simulink model "backstepping_and_CT"  (R2020b)
settings: Solver=ode23t  StartTime=0.0  StopTime=30  RelTol=1e-3
InitFcn:
  | parametersUR5_BACKSTEPPING
StopFcn:
  | show_results
values from neighbouring files (symbols this model uses):
  init_config = [0,-55.5,-131,-2.5,20,105]'*pi/180    [UR5_LI_SLOTINE.m]    (also in parametersUR5_ADAPTIVE_BACKSTEPPING.m = [0,-37,-110,-2.5,-1,55]'*pi/180; parametersUR5_BACKSTEPPING.m = [0,-37,-110,-2.5,-1,55]'*pi/180)
  m1 = ur5.links(1,1).m    [UR5_LI_SLOTINE.m]    (also in parametersUR5_ADAPTIVE_BACKSTEPPING.m; parametersUR5_BACKSTEPPING.m)
  m2 = ur5.links(1,2).m    [UR5_LI_SLOTINE.m]    (also in parametersUR5_ADAPTIVE_BACKSTEPPING.m; parametersUR5_BACKSTEPPING.m)
  m3 = ur5.links(1,3).m    [UR5_LI_SLOTINE.m]    (also in parametersUR5_ADAPTIVE_BACKSTEPPING.m; parametersUR5_BACKSTEPPING.m)
  m4 = ur5.links(1,4).m    [UR5_LI_SLOTINE.m]    (also in parametersUR5_ADAPTIVE_BACKSTEPPING.m; parametersUR5_BACKSTEPPING.m)
  m5 = ur5.links(1,5).m    [UR5_LI_SLOTINE.m]    (also in parametersUR5_ADAPTIVE_BACKSTEPPING.m; parametersUR5_BACKSTEPPING.m)
  m6 = ur5.links(1,6).m    [UR5_LI_SLOTINE.m]    (also in parametersUR5_ADAPTIVE_BACKSTEPPING.m; parametersUR5_BACKSTEPPING.m)
  Ts = 1/100    (= 0.01)    [UR5_LI_SLOTINE.m]    (also in parametersUR5_ADAPTIVE_BACKSTEPPING.m; parametersUR5_BACKSTEPPING.m)
libraries: simulink x2
settings Model: Creator=marym  LastModifiedBy=stefa
settings DebuggingCC: SFMachineParentedDataDiag=error

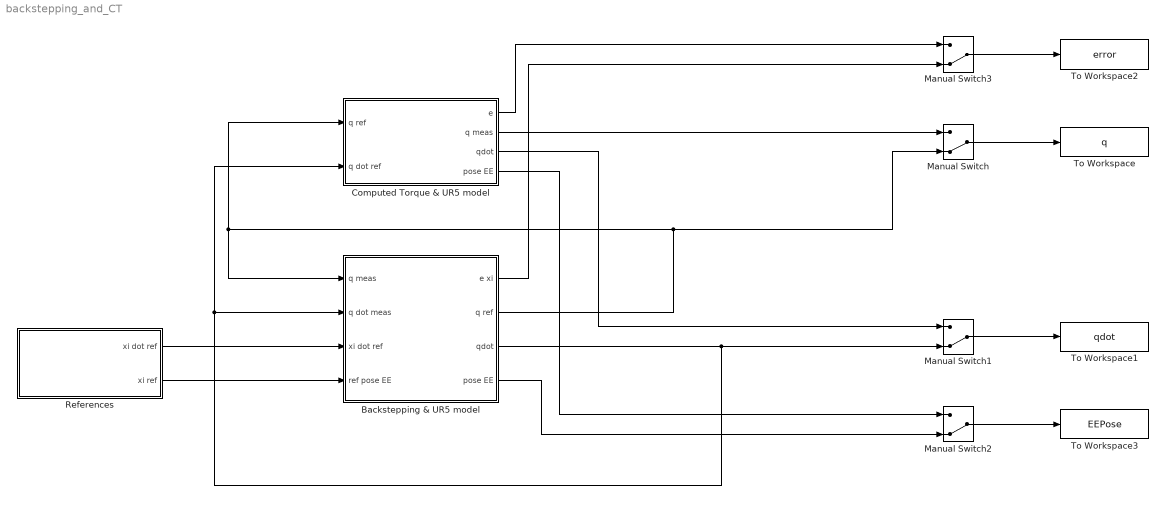
== system backstepping_and_CT ==
  Backstepping & UR5 model : Subsystem
  Computed Torque & UR5 model : Subsystem
  Manual Switch{,1..3} (4 alike) : ManualSwitch  CurrentSetting=0
  References : Subsystem
  To Workspace : ToWorkspace  VariableName=q  SaveFormat=Timeseries  SampleTime=Ts
  To Workspace1 : ToWorkspace  VariableName=qdot  SaveFormat=Timeseries  SampleTime=Ts
  To Workspace2 : ToWorkspace  VariableName=error  SaveFormat=Timeseries  SampleTime=Ts
  To Workspace3 : ToWorkspace  VariableName=EEPose  SaveFormat=Timeseries  SampleTime=Ts
  wires:
  Manual Switch/1 -> To Workspace/1
  Manual Switch1/1 -> To Workspace1/1
  Manual Switch2/1 -> To Workspace3/1
  Manual Switch3/1 -> To Workspace2/1
  Backstepping & UR5 model/3(qdot) -> Computed Torque & UR5 model/2(q dot ref), Backstepping & UR5 model/2(q dot meas), Manual Switch1/2
  Backstepping & UR5 model/2(q ref) -> Manual Switch/2, Computed Torque & UR5 model/1(q ref), Backstepping & UR5 model/1(q meas)
  References/1(xi dot ref) -> Backstepping & UR5 model/3(xi dot ref)
  References/2(xi ref) -> Backstepping & UR5 model/4(ref pose EE)
  Backstepping & UR5 model/1(e xi) -> Manual Switch3/2
  Backstepping & UR5 model/4(pose EE) -> Manual Switch2/2
  Computed Torque & UR5 model/1(e) -> Manual Switch3/1
  Computed Torque & UR5 model/2(q meas) -> Manual Switch/1
  Computed Torque & UR5 model/3(qdot) -> Manual Switch1/1
  Computed Torque & UR5 model/4(pose EE) -> Manual Switch2/1

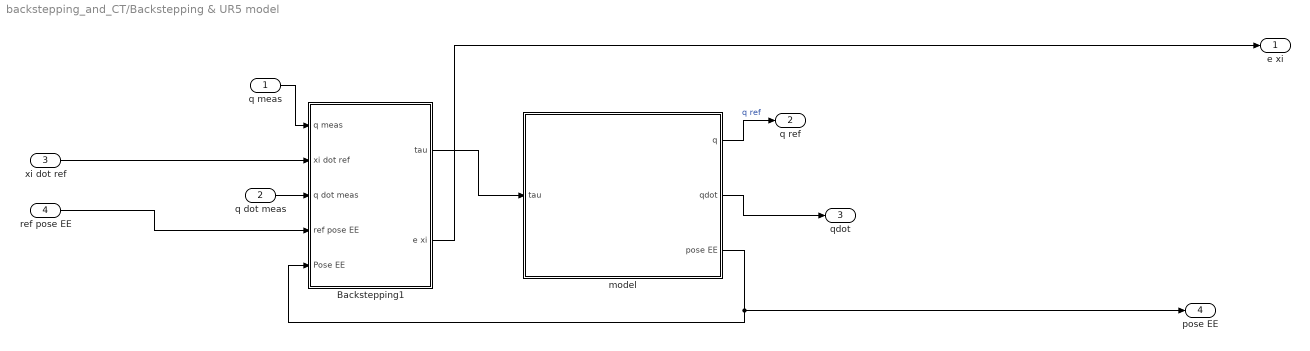
== system backstepping_and_CT/Backstepping & UR5 model ==
  q meas : Inport
  q dot meas : Inport  Port=2
  xi dot ref : Inport  Port=3
  ref pose EE : Inport  Port=4
  Backstepping1 : Subsystem
  model : Subsystem
  e xi : Outport
  q ref : Outport  Port=2
  qdot : Outport  Port=3
  pose EE : Outport  Port=4
  wires:
  model/1(q) -> q ref/1  "q ref"
  Backstepping1/2(e xi) -> e xi/1
  ref pose EE/1 -> Backstepping1/4(ref pose EE)
  Backstepping1/1(tau) -> model/1(tau)
  model/3(pose EE) -> pose EE/1, Backstepping1/5(Pose EE)
  model/2(qdot) -> qdot/1
  q meas/1 -> Backstepping1/1(q meas)
  q dot meas/1 -> Backstepping1/3(q dot meas)
  xi dot ref/1 -> Backstepping1/2(xi dot ref)

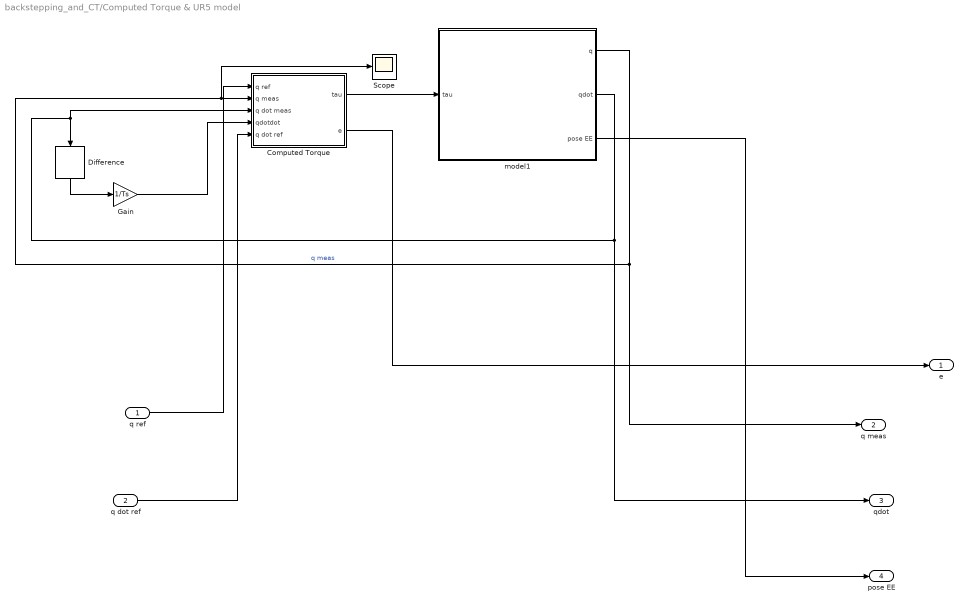
== system backstepping_and_CT/Computed Torque & UR5 model ==
  q ref : Inport
  q dot ref : Inport  Port=2
  Computed Torque : Subsystem
  Difference : simulink/Discrete/Difference  ICPrevInput=0.0  OutMin=[]  OutMax=[]  OutDataType=fixdt(1, 16)  OutScaling=2^-10  DoSatur=off
  Gain : Gain  Gain=1/Ts
  Scope : Scope
  model1 : Subsystem
  e : Outport
  q meas : Outport  Port=2
  qdot : Outport  Port=3
  pose EE : Outport  Port=4
  wires:
  model1/3(pose EE) -> pose EE/1
  model1/1(q) -> q meas/1, Scope/1, Computed Torque/2(q meas)  "q meas"
  Computed Torque/1(tau) -> model1/1(tau)
  model1/2(qdot) -> qdot/1, Computed Torque/3(q dot meas), Difference/1
  q ref/1 -> Computed Torque/1(q ref)
  Difference/1 -> Gain/1
  Gain/1 -> Computed Torque/4(qdotdot)
  q dot ref/1 -> Computed Torque/5(q dot ref)
  Computed Torque/2(e) -> e/1

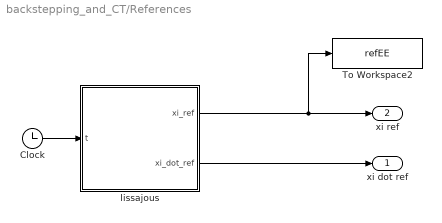
== system backstepping_and_CT/References ==
  Clock : Clock
  To Workspace2 : ToWorkspace  VariableName=refEE  SaveFormat=Timeseries  SampleTime=Ts
  lissajous : MATLAB Function  TreatAsAtomicUnit=on
  xi dot ref : Outport
  xi ref : Outport  Port=2
  wires:
  Clock/1 -> lissajous/1(t)
  lissajous/1(xi_ref) -> To Workspace2/1, xi ref/1
  lissajous/2(xi_dot_ref) -> xi dot ref/1

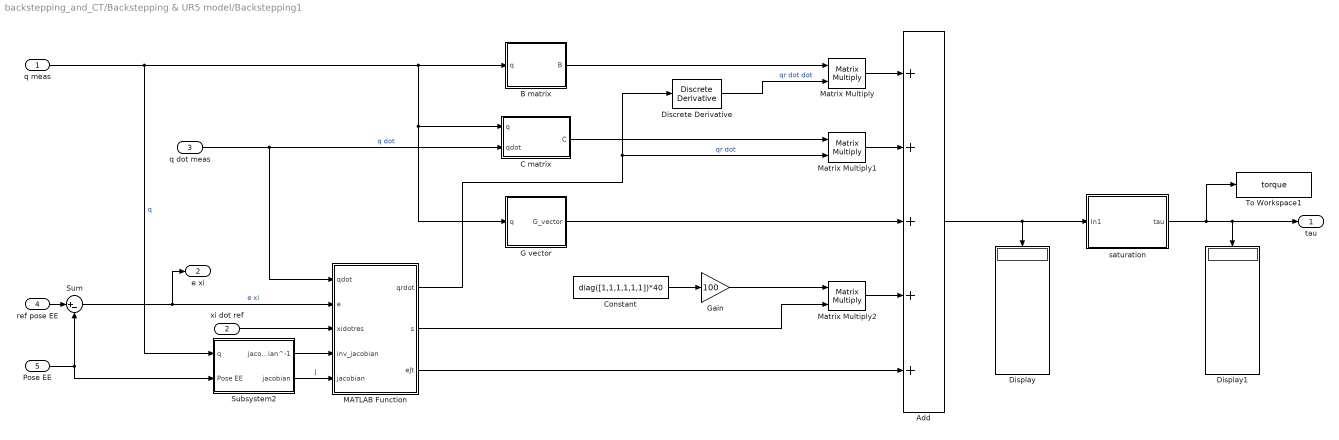
== system backstepping_and_CT/Backstepping & UR5 model/Backstepping1 ==
  q meas : Inport
  xi dot ref : Inport  Port=2
  q dot meas : Inport  Port=3
  ref pose EE : Inport  Port=4
  Pose EE : Inport  Port=5
  Add : Sum  Inputs=+++++
  B matrix : MATLAB Function  TreatAsAtomicUnit=on
  C matrix : MATLAB Function  TreatAsAtomicUnit=on
  Constant : Constant  Value=diag([1,1,1,1,1,1])*40
  Discrete Derivative : simulink/Discrete/Discrete Derivative  gainval=1.0  ICPrevScaledInput=0.0  OutMin=[]  OutMax=[]  OutDataType=fixdt(1, 16)  OutScaling=2^-10  DoSatur=off
  Display : Display
  Display1 : Display
  G vector : MATLAB Function  TreatAsAtomicUnit=on
  Gain : Gain  Gain=100
  MATLAB Function : MATLAB Function  TreatAsAtomicUnit=on
  Matrix Multiply : Product  Multiplication=Matrix(*)
  Matrix Multiply1 : Product  Multiplication=Matrix(*)
  Matrix Multiply2 : Product  Multiplication=Matrix(*)
  Subsystem2 : Subsystem
  Sum : Sum  Inputs=|+-
  To Workspace1 : ToWorkspace  VariableName=torque  SaveFormat=Timeseries  SampleTime=Ts
  saturation : Subsystem
  tau : Outport
  e xi : Outport  Port=2
  wires:
  Add/1 -> Display/1, saturation/1(In1)
  Matrix Multiply/1 -> Add/1
  Matrix Multiply1/1 -> Add/2
  B matrix/1(B) -> Matrix Multiply/1
  C matrix/1(C) -> Matrix Multiply1/1
  q meas/1 -> G vector/1(q), C matrix/1(q), B matrix/1(q), Subsystem2/1(q)  "q"
  G vector/1(G_vector) -> Add/3
  Discrete Derivative/1 -> Matrix Multiply/2  "qr dot dot"
  MATLAB Function/1(qrdot) -> Matrix Multiply1/2, Discrete Derivative/1  "qr dot"
  q dot meas/1 -> MATLAB Function/1(qdot), C matrix/2(qdot)  "q dot"
  ref pose EE/1 -> Sum/1
  Pose EE/1 -> Sum/2, Subsystem2/2(Pose EE)
  Sum/1 -> e xi/1, MATLAB Function/2(e)  "e xi"
  Subsystem2/1(jacobian^-1) -> MATLAB Function/4(inv_jacobian)
  MATLAB Function/3(eJt) -> Add/5
  Subsystem2/2(jacobian) -> MATLAB Function/5(jacobian)  "J"
  MATLAB Function/2(s) -> Matrix Multiply2/2
  Matrix Multiply2/1 -> Add/4
  Constant/1 -> Gain/1
  xi dot ref/1 -> MATLAB Function/3(xidotres)
  Gain/1 -> Matrix Multiply2/1
  saturation/1(tau) -> tau/1, Display1/1, To Workspace1/1

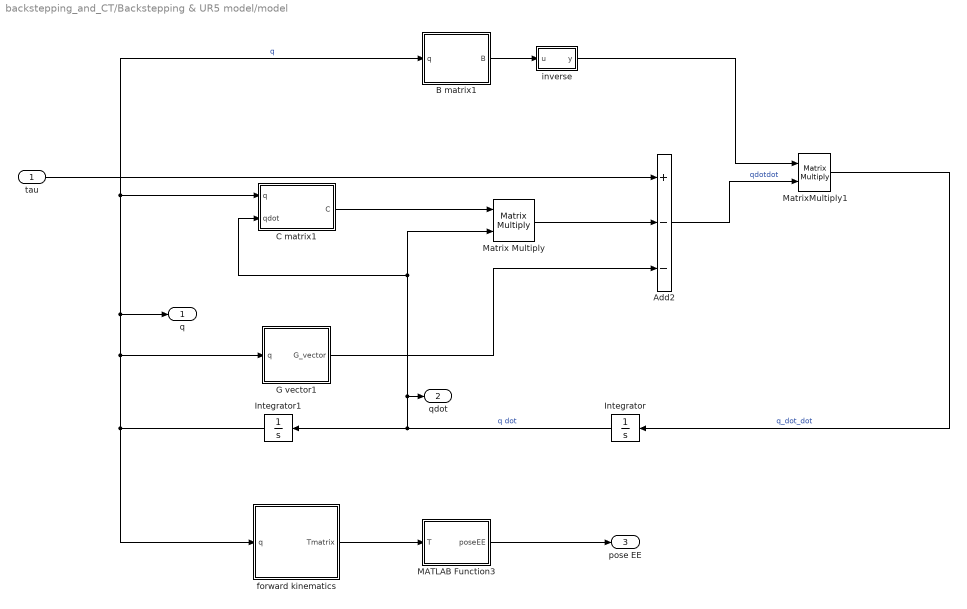
== system backstepping_and_CT/Backstepping & UR5 model/model ==
  tau : Inport
  Add2 : Sum  Inputs=+--
  B matrix1 : MATLAB Function  TreatAsAtomicUnit=on
  C matrix1 : MATLAB Function  TreatAsAtomicUnit=on
  G vector1 : MATLAB Function  TreatAsAtomicUnit=on
  Integrator : Integrator  InitialCondition=[0,0,0,0,0,0]'
  Integrator1 : Integrator  InitialCondition=init_config
  MATLAB Function3 : MATLAB Function  TreatAsAtomicUnit=on
  Matrix Multiply : Product  Multiplication=Matrix(*)
  MatrixMultiply1 : Product  Multiplication=Matrix(*)
  forward kinematics : MATLAB Function  TreatAsAtomicUnit=on
  inverse : MATLAB Function  TreatAsAtomicUnit=on
  q : Outport
  qdot : Outport  Port=2
  pose EE : Outport  Port=3
  wires:
  MatrixMultiply1/1 -> Integrator/1  "q_dot_dot"
  B matrix1/1(B) -> inverse/1(u)
  inverse/1(y) -> MatrixMultiply1/1
  tau/1 -> Add2/1
  Matrix Multiply/1 -> Add2/2
  C matrix1/1(C) -> Matrix Multiply/1
  Integrator/1 -> C matrix1/2(qdot), Matrix Multiply/2, qdot/1, Integrator1/1  "q dot"
  Integrator1/1 -> forward kinematics/1(q), G vector1/1(q), q/1, B matrix1/1(q), C matrix1/1(q)  "q"
  G vector1/1(G_vector) -> Add2/3
  Add2/1 -> MatrixMultiply1/2  "qdotdot"
  forward kinematics/1(Tmatrix) -> MATLAB Function3/1(T)
  MATLAB Function3/1(poseEE) -> pose EE/1

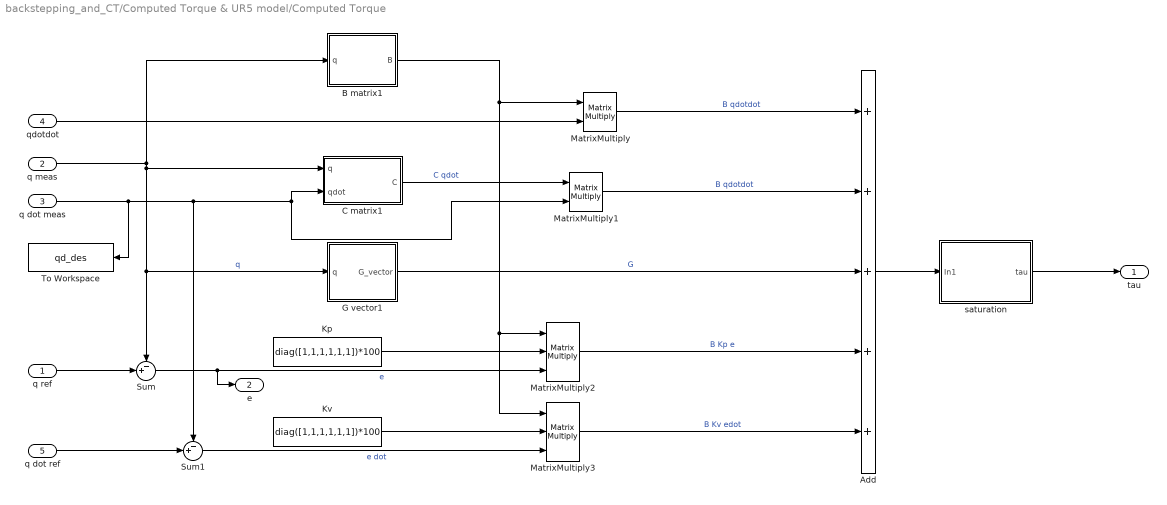
== system backstepping_and_CT/Computed Torque & UR5 model/Computed Torque ==
  q ref : Inport
  q meas : Inport  Port=2
  q dot meas : Inport  Port=3
  qdotdot : Inport  Port=4
  q dot ref : Inport  Port=5
  Add : Sum  Inputs=+++++
  B matrix1 : MATLAB Function  TreatAsAtomicUnit=on
  C matrix1 : MATLAB Function  TreatAsAtomicUnit=on
  G vector1 : MATLAB Function  TreatAsAtomicUnit=on
  Kp : Constant  Value=diag([1,1,1,1,1,1])*100
  Kv : Constant  Value=diag([1,1,1,1,1,1])*100
  MatrixMultiply : Product  Multiplication=Matrix(*)
  MatrixMultiply1 : Product  Multiplication=Matrix(*)
  MatrixMultiply2 : Product  Inputs=3  Multiplication=Matrix(*)
  MatrixMultiply3 : Product  Inputs=3  Multiplication=Matrix(*)
  Sum : Sum  Inputs=-+|
  Sum1 : Sum  Inputs=-+|
  To Workspace : ToWorkspace  VariableName=qd_des  SaveFormat=Timeseries  SampleTime=-1
  saturation : Subsystem
  tau : Outport
  e : Outport  Port=2
  wires:
  q meas/1 -> C matrix1/1(q), G vector1/1(q), Sum/1, B matrix1/1(q)  "q"
  MatrixMultiply/1 -> Add/1  "B qdotdot"
  B matrix1/1(B) -> MatrixMultiply3/1, MatrixMultiply2/1, MatrixMultiply/1
  q dot meas/1 -> To Workspace/1, Sum1/1, C matrix1/2(qdot), MatrixMultiply1/2
  C matrix1/1(C) -> MatrixMultiply1/1  "C qdot"
  G vector1/1(G_vector) -> Add/3  "G"
  q ref/1 -> Sum/2
  Sum/1 -> e/1, MatrixMultiply2/3  "e"
  MatrixMultiply2/1 -> Add/4  "B Kp e"
  q dot ref/1 -> Sum1/2
  Sum1/1 -> MatrixMultiply3/3  "e dot"
  MatrixMultiply3/1 -> Add/5  "B Kv edot"
  Kp/1 -> MatrixMultiply2/2
  Kv/1 -> MatrixMultiply3/2
  qdotdot/1 -> MatrixMultiply/2
  MatrixMultiply1/1 -> Add/2  "B qdotdot"
  Add/1 -> saturation/1(In1)
  saturation/1(tau) -> tau/1

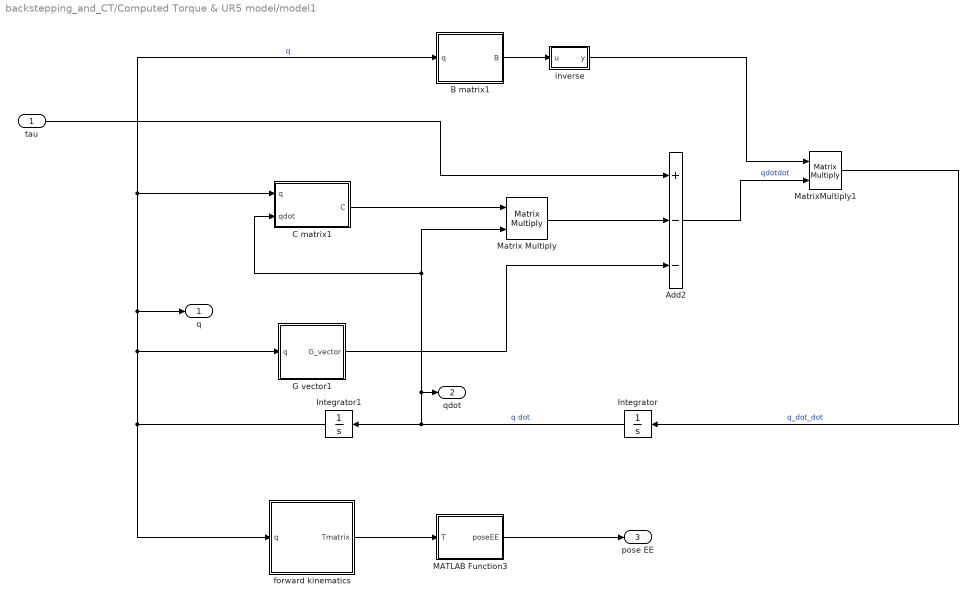
== system backstepping_and_CT/Computed Torque & UR5 model/model1 ==
  tau : Inport
  Add2 : Sum  Inputs=+--
  B matrix1 : MATLAB Function  TreatAsAtomicUnit=on
  C matrix1 : MATLAB Function  TreatAsAtomicUnit=on
  G vector1 : MATLAB Function  TreatAsAtomicUnit=on
  Integrator : Integrator  InitialCondition=[0,0,0,0,0,0]'
  Integrator1 : Integrator  InitialCondition=init_config
  MATLAB Function3 : MATLAB Function  TreatAsAtomicUnit=on
  Matrix Multiply : Product  Multiplication=Matrix(*)
  MatrixMultiply1 : Product  Multiplication=Matrix(*)
  forward kinematics : MATLAB Function  TreatAsAtomicUnit=on
  inverse : MATLAB Function  TreatAsAtomicUnit=on
  q : Outport
  qdot : Outport  Port=2
  pose EE : Outport  Port=3
  wires:
  MatrixMultiply1/1 -> Integrator/1  "q_dot_dot"
  B matrix1/1(B) -> inverse/1(u)
  inverse/1(y) -> MatrixMultiply1/1
  tau/1 -> Add2/1
  Matrix Multiply/1 -> Add2/2
  C matrix1/1(C) -> Matrix Multiply/1
  Integrator/1 -> C matrix1/2(qdot), Matrix Multiply/2, qdot/1, Integrator1/1  "q dot"
  Integrator1/1 -> G vector1/1(q), q/1, B matrix1/1(q), C matrix1/1(q), forward kinematics/1(q)  "q"
  G vector1/1(G_vector) -> Add2/3
  Add2/1 -> MatrixMultiply1/2  "qdotdot"
  forward kinematics/1(Tmatrix) -> MATLAB Function3/1(T)
  MATLAB Function3/1(poseEE) -> pose EE/1

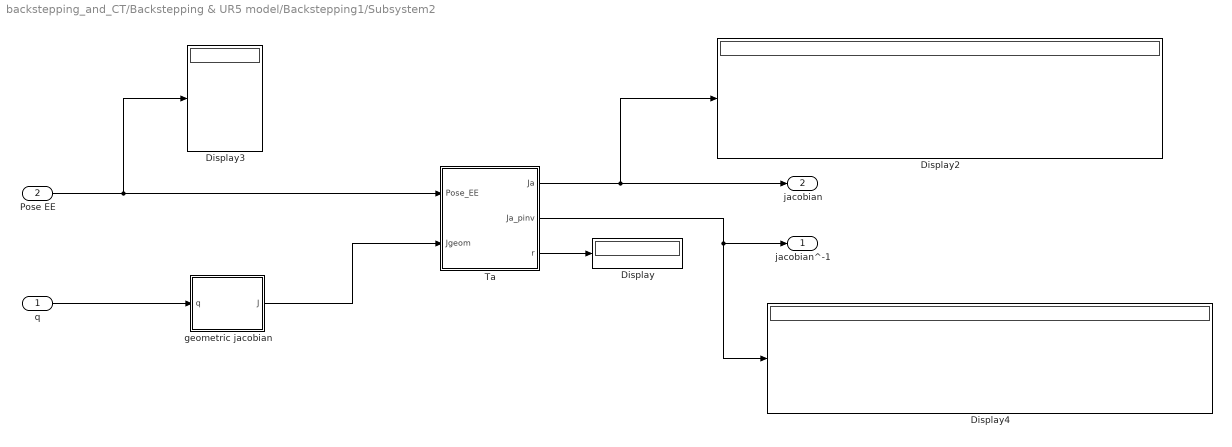
== system backstepping_and_CT/Backstepping & UR5 model/Backstepping1/Subsystem2 ==
  q : Inport
  Pose EE : Inport  Port=2
  Display{,2..4} (4 alike) : Display
  Ta : MATLAB Function  TreatAsAtomicUnit=on
  geometric jacobian : MATLAB Function  TreatAsAtomicUnit=on
  jacobian^-1 : Outport
  jacobian : Outport  Port=2
  wires:
  Pose EE/1 -> Ta/1(Pose_EE), Display3/1
  q/1 -> geometric jacobian/1(q)
  Ta/2(Ja_pinv) -> jacobian^-1/1, Display4/1
  Ta/1(Ja) -> jacobian/1, Display2/1
  Ta/3(r) -> Display/1
  geometric jacobian/1(J) -> Ta/2(Jgeom)

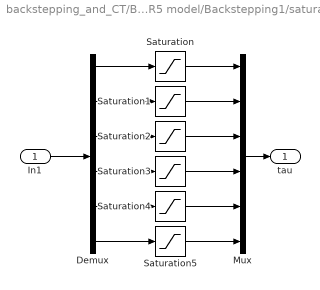
== system backstepping_and_CT/Backstepping & UR5 model/Backstepping1/saturation ==
  In1 : Inport
  Demux : Demux  Outputs=6
  Mux : Mux  Inputs=6
  Saturation : Saturate  UpperLimit=150  LowerLimit=-150
  Saturation1 : Saturate  UpperLimit=150  LowerLimit=-150
  Saturation2 : Saturate  UpperLimit=150  LowerLimit=-150
  Saturation3 : Saturate  UpperLimit=28  LowerLimit=-28
  Saturation4 : Saturate  UpperLimit=28  LowerLimit=-28
  Saturation5 : Saturate  UpperLimit=28  LowerLimit=-28
  tau : Outport
  wires:
  In1/1 -> Demux/1
  Mux/1 -> tau/1
  Demux/1 -> Saturation/1
  Demux/2 -> Saturation1/1
  Demux/3 -> Saturation2/1
  Demux/4 -> Saturation3/1
  Demux/5 -> Saturation4/1
  Demux/6 -> Saturation5/1
  Saturation/1 -> Mux/1
  Saturation1/1 -> Mux/2
  Saturation2/1 -> Mux/3
  Saturation3/1 -> Mux/4
  Saturation4/1 -> Mux/5
  Saturation5/1 -> Mux/6

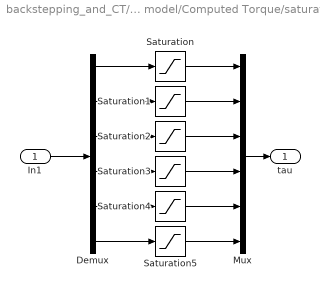
== system backstepping_and_CT/Computed Torque & UR5 model/Computed Torque/saturation ==
  In1 : Inport
  Demux : Demux  Outputs=6
  Mux : Mux  Inputs=6
  Saturation : Saturate  UpperLimit=150  LowerLimit=-150
  Saturation1 : Saturate  UpperLimit=150  LowerLimit=-150
  Saturation2 : Saturate  UpperLimit=150  LowerLimit=-150
  Saturation3 : Saturate  UpperLimit=28  LowerLimit=-28
  Saturation4 : Saturate  UpperLimit=28  LowerLimit=-28
  Saturation5 : Saturate  UpperLimit=28  LowerLimit=-28
  tau : Outport
  wires:
  In1/1 -> Demux/1
  Mux/1 -> tau/1
  Demux/1 -> Saturation/1
  Demux/2 -> Saturation1/1
  Demux/3 -> Saturation2/1
  Demux/4 -> Saturation3/1
  Demux/5 -> Saturation4/1
  Demux/6 -> Saturation5/1
  Saturation/1 -> Mux/1
  Saturation1/1 -> Mux/2
  Saturation2/1 -> Mux/3
  Saturation3/1 -> Mux/4
  Saturation4/1 -> Mux/5
  Saturation5/1 -> Mux/6

== matlab function backstepping_and_CT/Computed Torque & UR5 model/model1/MATLAB Function3 ==
  data: T input; poseEE output
function poseEE = fcn(T)
    poseEE = zeros(6,1);
    coder.extrinsic('tform2eul');
    
    O = [0; 0; 0];        % world origin frame

    position = T * [O; 1];
    orientation = tform2eul(T, 'ZYZ');

    poseEE = [position(1:3); orientation'];
end

== matlab function backstepping_and_CT/Backstepping & UR5 model/model/forward kinematics ==
  data: q input; Tmatrix output
function Tmatrix = fkine(q)
%#codegen

%    This function was generated by the Symbolic Math Toolbox version 8.6.
%    20-Jan-2022 14:28:01

q1 = q(1);
q2 = q(2);
q3 = q(3);
q4 = q(4);
q5 = q(5);
q6 = q(6);
t2 = cos(q1);
t3 = cos(q2);
t4 = cos(q3);
t5 = cos(q4);
t6 = cos(q5);
t7 = cos(q6);
t8 = sin(q1);
t9 = sin(q2);
t10 = sin(q3);
t11 = sin(q4);
t12 = sin(q5);
t13 = sin(q6);
t14 = q2+q3;
t23 = cos(1.570796327);
t24 = sin(1.570796327);
t25 = sin(3.141592654);
t15 = q4+t14;
t16 = t2.*t3;
t18 = t2.*t9;
t19 = t3.*t8;
t21 = t8.*t9;
t26 = t23.^2;
t27 = t24.^2;
t58 = t2.*t23.*t24;
t59 = t8.*t23.*t24;
t17 = cos(t15);
t20 = sin(t15);
t28 = t16.*t23;
t29 = t18.*t23;
t30 = t19.*t23;
t31 = t21.*t23;
t32 = t2.*t27;
t33 = t8.*t27;
t38 = t3.*t4.*t5.*t27;
t39 = t3.*t10.*t11.*t27;
t40 = t4.*t9.*t11.*t27;
t41 = t5.*t9.*t10.*t27;
t60 = -t58;
t22 = t17+1.0;
t34 = -t28;
t35 = -t31;
t36 = -t33;
t37 = t6.*t20.*t24;
t42 = -t38;
t43 = t18+t30;
t44 = t19+t29;
t61 = t12.*t20.*t23.*t24;
t45 = t16+t35;
t46 = t21+t34;
t47 = (t12.*t22.*t25)./2.0;
t48 = t4.*t43;
t49 = t4.*t44;
t50 = t10.*t43;
t51 = t10.*t44;
t62 = (t6.*t22.*t23.*t25)./2.0;
t85 = t26+t39+t40+t41+t42;
t52 = t4.*t45;
t53 = t4.*t46;
t54 = t10.*t45;
t55 = t10.*t46;
t56 = -t50;
t63 = -t62;
t64 = t37+t47;
t89 = t24.*t85;
t57 = -t55;
t65 = t48+t54;
t66 = t51+t53;
t68 = t52+t56;
t72 = -t5.*(t50-t52);
t80 = -t11.*t23.*(t50-t52);
t82 = -t11.*t24.*(t50-t52);
t103 = t61+t63+t89;
t67 = t49+t57;
t69 = t11.*t65;
t70 = t11.*t66;
t75 = t5.*t23.*t65;
t76 = t5.*t23.*t66;
t77 = t5.*t24.*t65;
t78 = t5.*t24.*t66;
t71 = t5.*t67;
t73 = -t69;
t74 = -t70;
t79 = t11.*t23.*t67;
t81 = t11.*t24.*t67;
t87 = -t6.*(t69+t5.*(t50-t52));
t91 = -t12.*t23.*(t69+t5.*(t50-t52));
t93 = t36+t75+t80;
t97 = t59+t77+t82;
t83 = t71+t74;
t84 = t72+t73;
t86 = -t6.*(t70-t71);
t88 = t6.*(t70-t71);
t90 = -t12.*t23.*(t70-t71);
t92 = t32+t76+t79;
t95 = t12.*t93;
t98 = t60+t78+t81;
t100 = t6.*t23.*t93;
t101 = t24.*t97;
t94 = t12.*t92;
t96 = -t95;
t99 = t6.*t23.*t92;
t102 = t24.*t98;
t107 = t91+t100+t101;
t104 = t88+t94;
t105 = t87+t96;
t106 = t90+t99+t102;
Tmatrix = reshape([-t13.*t107-t7.*(t95+t6.*(t69+t5.*(t50-t52))),-t7.*t104-t13.*t106,t7.*t64-t13.*t103,0.0,-t7.*t107+t13.*(t95+t6.*(t69+t5.*(t50-t52))),-t7.*t106+t13.*t104,-t13.*t64-t7.*t103,0.0,t23.*t97+t12.*t24.*(t69+t5.*(t50-t52))-t6.*t24.*t93,t23.*t98-t6.*t24.*t92+t12.*t24.*(t70-t71),t23.*t85-t12.*t20.*t27+(t6.*t22.*t24.*t25)./2.0,0.0,t16.*(-1.7e+1./4.0e+1)+t31.*(1.7e+1./4.0e+1)+t50.*3.9225e-1-t52.*3.9225e-1+t59.*9.465e-2+t77.*9.465e-2+t8.*t24.*1.0915e-1+t23.*t97.*8.23e-2+t12.*t24.*(t69+t5.*(t50-t52)).*8.23e-2-t6.*t24.*t93.*8.23e-2-t11.*t24.*(t50-t52).*9.465e-2,t19.*(-1.7e+1./4.0e+1)-t29.*(1.7e+1./4.0e+1)-t49.*3.9225e-1+t55.*3.9225e-1-t58.*9.465e-2+t78.*9.465e-2+t81.*9.465e-2-t2.*t24.*1.0915e-1+t23.*t98.*8.23e-2-t6.*t24.*t92.*8.23e-2+t12.*t24.*(t70-t71).*8.23e-2,t23.*1.0915e-1+t26.*9.465e-2-t9.*t24.*(1.7e+1./4.0e+1)-t23.*t38.*8.23e-2+t23.*t39.*8.23e-2+t23.*t40.*8.23e-2+t23.*t41.*8.23e-2+t23.^3.*8.23e-2-t5.*t27.*cos(t14).*9.465e-2+t11.*t27.*sin(t14).*9.465e-2-t3.*t10.*t24.*3.9225e-1-t4.*t9.*t24.*3.9225e-1+t6.*t24.*t25.*4.115e-2-t12.*t20.*t27.*8.23e-2+t6.*t17.*t24.*t25.*4.115e-2+8.9459e-2,1.0],[4,4]);

== matlab function backstepping_and_CT/Backstepping & UR5 model/Backstepping1/Subsystem2/Ta ==
  data: Pose_EE input; Ja output; Ja_pinv output; Jgeom input; r output
function [Ja, Ja_pinv, r ]= fcn(Pose_EE, Jgeom)
Ja=zeros(6,6);
Ja_pinv=zeros(6,6);

phi = Pose_EE(4);
theta = Pose_EE(5);

%% con ZYZ
Ta = [0     -sin(phi)       cos(phi)*sin(theta) ;
      0      cos(phi)       sin(phi)*sin(theta) ;
      1          0                    cos(theta)];


Ja = inv([eye(3), zeros(3); zeros(3), Ta]) * Jgeom;

%Ja_pinv = inv(Ja);
Ja_pinv = pinv(Ja, 0.0005);
%Ja_pinv = damped_pseudo_inverse(Ja,0.1,0.1);
r = rank(Ja);

end

== matlab function backstepping_and_CT/Computed Torque & UR5 model/model1/forward kinematics ==
  data: q input; Tmatrix output
function Tmatrix = fkine(q)
%#codegen

%    This function was generated by the Symbolic Math Toolbox version 8.6.
%    20-Jan-2022 14:28:01

q1 = q(1);
q2 = q(2);
q3 = q(3);
q4 = q(4);
q5 = q(5);
q6 = q(6);
t2 = cos(q1);
t3 = cos(q2);
t4 = cos(q3);
t5 = cos(q4);
t6 = cos(q5);
t7 = cos(q6);
t8 = sin(q1);
t9 = sin(q2);
t10 = sin(q3);
t11 = sin(q4);
t12 = sin(q5);
t13 = sin(q6);
t14 = q2+q3;
t23 = cos(1.570796327);
t24 = sin(1.570796327);
t25 = sin(3.141592654);
t15 = q4+t14;
t16 = t2.*t3;
t18 = t2.*t9;
t19 = t3.*t8;
t21 = t8.*t9;
t26 = t23.^2;
t27 = t24.^2;
t58 = t2.*t23.*t24;
t59 = t8.*t23.*t24;
t17 = cos(t15);
t20 = sin(t15);
t28 = t16.*t23;
t29 = t18.*t23;
t30 = t19.*t23;
t31 = t21.*t23;
t32 = t2.*t27;
t33 = t8.*t27;
t38 = t3.*t4.*t5.*t27;
t39 = t3.*t10.*t11.*t27;
t40 = t4.*t9.*t11.*t27;
t41 = t5.*t9.*t10.*t27;
t60 = -t58;
t22 = t17+1.0;
t34 = -t28;
t35 = -t31;
t36 = -t33;
t37 = t6.*t20.*t24;
t42 = -t38;
t43 = t18+t30;
t44 = t19+t29;
t61 = t12.*t20.*t23.*t24;
t45 = t16+t35;
t46 = t21+t34;
t47 = (t12.*t22.*t25)./2.0;
t48 = t4.*t43;
t49 = t4.*t44;
t50 = t10.*t43;
t51 = t10.*t44;
t62 = (t6.*t22.*t23.*t25)./2.0;
t85 = t26+t39+t40+t41+t42;
t52 = t4.*t45;
t53 = t4.*t46;
t54 = t10.*t45;
t55 = t10.*t46;
t56 = -t50;
t63 = -t62;
t64 = t37+t47;
t89 = t24.*t85;
t57 = -t55;
t65 = t48+t54;
t66 = t51+t53;
t68 = t52+t56;
t72 = -t5.*(t50-t52);
t80 = -t11.*t23.*(t50-t52);
t82 = -t11.*t24.*(t50-t52);
t103 = t61+t63+t89;
t67 = t49+t57;
t69 = t11.*t65;
t70 = t11.*t66;
t75 = t5.*t23.*t65;
t76 = t5.*t23.*t66;
t77 = t5.*t24.*t65;
t78 = t5.*t24.*t66;
t71 = t5.*t67;
t73 = -t69;
t74 = -t70;
t79 = t11.*t23.*t67;
t81 = t11.*t24.*t67;
t87 = -t6.*(t69+t5.*(t50-t52));
t91 = -t12.*t23.*(t69+t5.*(t50-t52));
t93 = t36+t75+t80;
t97 = t59+t77+t82;
t83 = t71+t74;
t84 = t72+t73;
t86 = -t6.*(t70-t71);
t88 = t6.*(t70-t71);
t90 = -t12.*t23.*(t70-t71);
t92 = t32+t76+t79;
t95 = t12.*t93;
t98 = t60+t78+t81;
t100 = t6.*t23.*t93;
t101 = t24.*t97;
t94 = t12.*t92;
t96 = -t95;
t99 = t6.*t23.*t92;
t102 = t24.*t98;
t107 = t91+t100+t101;
t104 = t88+t94;
t105 = t87+t96;
t106 = t90+t99+t102;
Tmatrix = reshape([-t13.*t107-t7.*(t95+t6.*(t69+t5.*(t50-t52))),-t7.*t104-t13.*t106,t7.*t64-t13.*t103,0.0,-t7.*t107+t13.*(t95+t6.*(t69+t5.*(t50-t52))),-t7.*t106+t13.*t104,-t13.*t64-t7.*t103,0.0,t23.*t97+t12.*t24.*(t69+t5.*(t50-t52))-t6.*t24.*t93,t23.*t98-t6.*t24.*t92+t12.*t24.*(t70-t71),t23.*t85-t12.*t20.*t27+(t6.*t22.*t24.*t25)./2.0,0.0,t16.*(-1.7e+1./4.0e+1)+t31.*(1.7e+1./4.0e+1)+t50.*3.9225e-1-t52.*3.9225e-1+t59.*9.465e-2+t77.*9.465e-2+t8.*t24.*1.0915e-1+t23.*t97.*8.23e-2+t12.*t24.*(t69+t5.*(t50-t52)).*8.23e-2-t6.*t24.*t93.*8.23e-2-t11.*t24.*(t50-t52).*9.465e-2,t19.*(-1.7e+1./4.0e+1)-t29.*(1.7e+1./4.0e+1)-t49.*3.9225e-1+t55.*3.9225e-1-t58.*9.465e-2+t78.*9.465e-2+t81.*9.465e-2-t2.*t24.*1.0915e-1+t23.*t98.*8.23e-2-t6.*t24.*t92.*8.23e-2+t12.*t24.*(t70-t71).*8.23e-2,t23.*1.0915e-1+t26.*9.465e-2-t9.*t24.*(1.7e+1./4.0e+1)-t23.*t38.*8.23e-2+t23.*t39.*8.23e-2+t23.*t40.*8.23e-2+t23.*t41.*8.23e-2+t23.^3.*8.23e-2-t5.*t27.*cos(t14).*9.465e-2+t11.*t27.*sin(t14).*9.465e-2-t3.*t10.*t24.*3.9225e-1-t4.*t9.*t24.*3.9225e-1+t6.*t24.*t25.*4.115e-2-t12.*t20.*t27.*8.23e-2+t6.*t17.*t24.*t25.*4.115e-2+8.9459e-2,1.0],[4,4]);

== matlab function backstepping_and_CT/Computed Torque & UR5 model/model1/inverse ==
  data: u input; y output
function y = fcn(u)

y = inv(u);

== matlab function backstepping_and_CT/Computed Torque & UR5 model/Computed Torque/B matrix1 ==
  data: q input; B output; m1 parameter; m2 parameter; m3 parameter; m4 parameter; m5 parameter; m6 parameter
function B = fcn(q, m1, m2, m3, m4, m5, m6)

B = Mmatrix(m1,m2,m3,m4,m5,m6,q(2),q(3),q(4),q(5));

== matlab function backstepping_and_CT/Computed Torque & UR5 model/Computed Torque/C matrix1 ==
  data: q input; C output; qdot input; m2 parameter; m3 parameter; m4 parameter; m5 parameter; m6 parameter
function C = C_matrix(q, qdot, m2, m3, m4, m5, m6)

C = Cmatrix(m2,m3,m4,m5,m6,q(2),q(3),q(4),q(5),qdot(1),qdot(2),qdot(3),qdot(4),qdot(5),qdot(6));

== matlab function backstepping_and_CT/Computed Torque & UR5 model/Computed Torque/G vector1 ==
  data: q input; G_vector output; m2 parameter; m3 parameter; m4 parameter; m5 parameter; m6 parameter
function G_vector = gravload(q, m2, m3, m4, m5, m6)

G_vector = Gvector(m2,m3,m4,m5,m6,q(2),q(3),q(4),q(5))';

== matlab function backstepping_and_CT/Backstepping & UR5 model/model/B matrix1 ==
  data: q input; B output; m1 parameter; m2 parameter; m3 parameter; m4 parameter; m5 parameter; m6 parameter
function B = fcn(q, m1, m2, m3, m4, m5, m6)

B = Mmatrix(m1,m2,m3,m4,m5,m6,q(2),q(3),q(4),q(5));

== matlab function backstepping_and_CT/Backstepping & UR5 model/model/C matrix1 ==
  data: q input; C output; qdot input; m2 parameter; m3 parameter; m4 parameter; m5 parameter; m6 parameter
function C = C_matrix(q, qdot, m2, m3, m4, m5, m6)

C = Cmatrix(m2,m3,m4,m5,m6,q(2),q(3),q(4),q(5),qdot(1),qdot(2),qdot(3),qdot(4),qdot(5),qdot(6));

== matlab function backstepping_and_CT/Backstepping & UR5 model/model/inverse ==
  data: u input; y output
function y = fcn(u)

y = inv(u);

== matlab function backstepping_and_CT/Backstepping & UR5 model/Backstepping1/B matrix ==
  data: q input; B output; m1 parameter; m2 parameter; m3 parameter; m4 parameter; m5 parameter; m6 parameter
function B = fcn(q, m1, m2, m3, m4, m5, m6)

B = Mmatrix(m1,m2,m3,m4,m5,m6,q(2),q(3),q(4),q(5));

== matlab function backstepping_and_CT/Backstepping & UR5 model/Backstepping1/Subsystem2/geometric jacobian ==
  data: q input; J output
function J = jacob0(q)

J = Jacobian0(q(1),q(2),q(3),q(4),q(5),q(6));

== matlab function backstepping_and_CT/Backstepping & UR5 model/model/MATLAB Function3 ==
  data: T input; poseEE output
function poseEE = fcn(T)
    poseEE = zeros(6,1);
    coder.extrinsic('tform2eul');
    
    O = [0; 0; 0];        % world origin frame

    position = T * [O; 1];
    orientation = tform2eul(T, 'ZYZ');

    poseEE = [position(1:3); orientation'];
end

== matlab function backstepping_and_CT/References/lissajous ==
  data: t input; xi_ref output; xi_dot_ref output
function [xi_ref,xi_dot_ref] = fcn(t)
    xi_ref = zeros(6,1);
    xi_dot_ref = zeros(6,1);

    initial_position = [-0.0597   -0.1914    0.6397];
    initial_orientation = [1.5558   -1.5797    3.0630]';
    A =0.15;
    metodo_di_slow = 0.1;
    p = 3;
    q = 2;
    
    x = A*sin(p*t*metodo_di_slow +pi/2) + initial_position(1)-A;
    y = initial_position(2);
    z = A*sin(q*t*metodo_di_slow ) + initial_position(3);
    
    xdot = -p*A*sin(p*t*metodo_di_slow )*metodo_di_slow ;
    ydot = 0;
    zdot = q*A * cos(q*t*metodo_di_slow )*metodo_di_slow ;
    
    position_ref = [x,y,z]';
    position_dot_ref =[xdot, ydot, zdot]';
    
    xi_ref = [position_ref ; initial_orientation];
    xi_dot_ref = [position_dot_ref ; 0;    0  ; 0];

== matlab function backstepping_and_CT/Backstepping & UR5 model/model/G vector1 ==
  data: q input; G_vector output; m2 parameter; m3 parameter; m4 parameter; m5 parameter; m6 parameter
function G_vector = gravload(q, m2, m3, m4, m5, m6)

G_vector = Gvector(m2,m3,m4,m5,m6,q(2),q(3),q(4),q(5))';

== matlab function backstepping_and_CT/Computed Torque & UR5 model/model1/B matrix1 ==
  data: q input; B output; m1 parameter; m2 parameter; m3 parameter; m4 parameter; m5 parameter; m6 parameter
function B = fcn(q, m1, m2, m3, m4, m5, m6)

B = Mmatrix(m1,m2,m3,m4,m5,m6,q(2),q(3),q(4),q(5));

== matlab function backstepping_and_CT/Backstepping & UR5 model/Backstepping1/C matrix ==
  data: q input; C output; qdot input; m2 parameter; m3 parameter; m4 parameter; m5 parameter; m6 parameter
function C = C_matrix(q, qdot, m2, m3, m4, m5, m6)

C = Cmatrix(m2,m3,m4,m5,m6,q(2),q(3),q(4),q(5),qdot(1),qdot(2),qdot(3),qdot(4),qdot(5),qdot(6));

== matlab function backstepping_and_CT/Backstepping & UR5 model/Backstepping1/G vector ==
  data: q input; G_vector output; m2 parameter; m3 parameter; m4 parameter; m5 parameter; m6 parameter
function G_vector = gravload(q, m2, m3, m4, m5, m6)

G_vector = Gvector(m2,m3,m4,m5,m6,q(2),q(3),q(4),q(5))';

== matlab function backstepping_and_CT/Backstepping & UR5 model/Backstepping1/MATLAB Function ==
  data: qdot input; e input; qrdot output; s output; xidotres input; inv_jacobian input; jacobian input; eJt output
function [qrdot, s, eJt] = fcn(qdot, e, xidotres, inv_jacobian, jacobian)
%#codegen


%lambda =0.1*diag([1,1,1,0.1,0.1,0.1]); ultimo
lambda =50*diag([1,1,1,0.1,0.01,0.7]);

edot = xidotres - jacobian*(qdot);

s = inv_jacobian * (edot + lambda * e);

qrdot = s + qdot;

% gain = 1*diag([1,1,1,0.01,0.01,0.01]);

eJt = jacobian'*e;

== matlab function backstepping_and_CT/Computed Torque & UR5 model/model1/C matrix1 ==
  data: q input; C output; qdot input; m2 parameter; m3 parameter; m4 parameter; m5 parameter; m6 parameter
function C = C_matrix(q, qdot, m2, m3, m4, m5, m6)

C = Cmatrix(m2,m3,m4,m5,m6,q(2),q(3),q(4),q(5),qdot(1),qdot(2),qdot(3),qdot(4),qdot(5),qdot(6));

== matlab function backstepping_and_CT/Computed Torque & UR5 model/model1/G vector1 ==
  data: q input; G_vector output; m2 parameter; m3 parameter; m4 parameter; m5 parameter; m6 parameter
function G_vector = gravload(q, m2, m3, m4, m5, m6)

G_vector = Gvector(m2,m3,m4,m5,m6,q(2),q(3),q(4),q(5))';
